simulink model "Goto_From"  (R2023b)
settings: Solver=VariableStepAuto  StartTime=0.0  StopTime=10.0  RelTol=1e-3
libraries: simulink x1
settings Model: Creator=hp  LastModifiedBy=hp

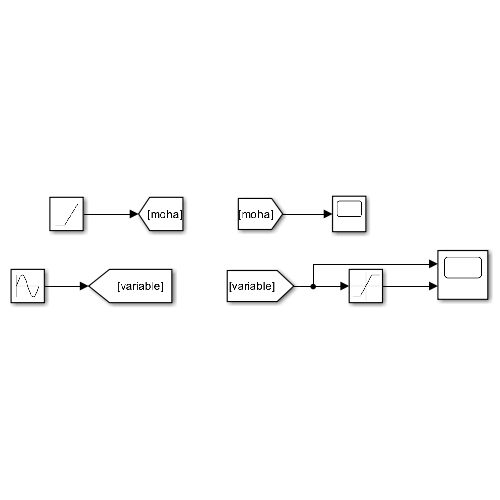
[thumbnail: Simulink's stored preview of the top-level diagram]
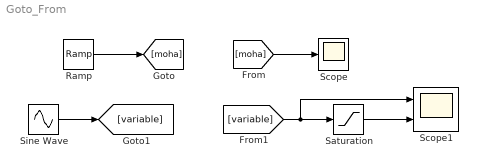
== system Goto_From ==
  Ramp : simulink/Sources/Ramp  slope=1  start=0  InitialOutput=0
  Saturation : Saturate
  Scope : Scope
  Scope1 : Scope  NumInputPorts=2
  Sine Wave : Sin  SampleTime=0
  wires:
  Ramp/1 -> [moha]
  [moha] -> Scope/1
  Sine Wave/1 -> [variable]
  [variable] -> Scope1/1, Saturation/1
  Saturation/1 -> Scope1/2
